simulink model "AutoMotive"  (R2020b)
settings: Solver=VariableStepAuto  StartTime=0.0  StopTime=10.0  RelTol=1e-3
settings Model: Creator=99003759  LastModifiedBy=99003759

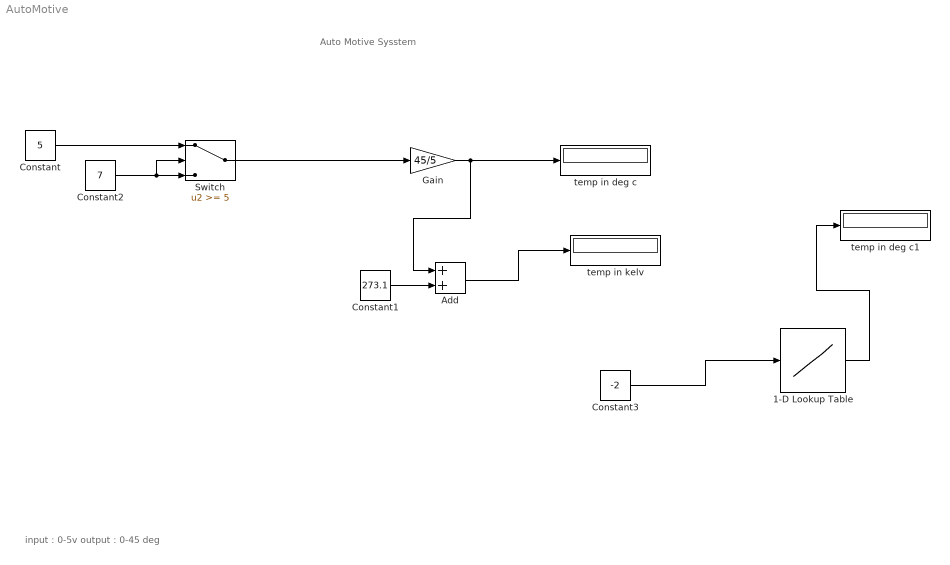
== system AutoMotive ==
  note: input : 0-5v
      | output : 0-45 deg
  note: Auto Motive Sysstem
  1-D Lookup Table : Lookup_n-D  NumberOfTableDimensions=1  BreakpointsForDimension1=[0:0.01:5]  Table=[0:0.09:45]  ExtrapMethod=Clip  UseLastTableValue=on  InternalRulePriority=Speed  RndMeth=Simplest  InputSameDT=on
  Add : Sum
  Constant : Constant  Value=5
  Constant1 : Constant  Value=273.1
  Constant2 : Constant  Value=7
  Constant3 : Constant  Value=-2
  Gain : Gain  Gain=45/5
  Switch : Switch  Threshold=5
  temp in deg c : Display
  temp in deg c1 : Display
  temp in kelv : Display
  wires:
  Gain/1 -> Add/1, temp in deg c/1
  Constant1/1 -> Add/2
  Add/1 -> temp in kelv/1
  Constant/1 -> Switch/1
  Switch/1 -> Gain/1
  Constant2/1 -> Switch/2, Switch/3
  Constant3/1 -> 1-D Lookup Table/1
  1-D Lookup Table/1 -> temp in deg c1/1
